simulink model "mpc_swarm_5"  (R2026a)
settings: Solver=ode4  FixedStep=0.004
undefined symbols (not defined in the file or in its folder): controlParams, eQ, eT, GravityAcc, kQ, kT, Mass, minPWM, mpc_swarm_step, rotorsSpeedDown, rotorsSpeedUp, SampleTime, uavParam
libraries: slpidlib x120, simulink x55, robotcorelib x20, matrix_library x20, aerolibasang x20, aerolibobsolete x5, uavutilslib x5
(part 5 of 14)

== system mpc_swarm_5/drone_1/pid_velocity/Subsystem ==
  roll_des : Inport
  pitch_des : Inport  Port=2
  yaw_des : Inport  Port=3
  euler_act : Inport  Port=4
  "[pqr_act" : Inport  Port=5
  Constant24 : Constant  Value=2
  Constant25 : Constant  Value=2
  Constant26 : Constant  Value=3
  Constant27 : Constant  Value=3
  Constant{30..31,35..36,42} (5 alike) : Constant  Value=0.01
  Constant32 : Constant  Value=10
  Constant33 : Constant
  Constant34 : Constant  Value=3
  Constant38 : Constant  Value=10
  Constant39 : Constant
  Constant40 : Constant  Value=5
  Constant41 : Constant  Value=0.1
  Constant49 : Constant  Value=10
  Constant50 : Constant  Value=2
  Constant7 : Constant  Value=0  OutDataTypeStr=boolean
  Demux1 : Demux  Outputs=3
  Demux5 : Demux  Outputs=3
  Gain10 : Gain  Gain=-1
  Gain11 : Gain  Gain=-1
  Gain9 : Gain  Gain=-1
  Mux : Mux  Inputs=3
  Mux4 : Mux  Inputs=3
  PID Controller3 : slpidlib/PID Controller  Controller=P  Form=Parallel  TimeDomain=Discrete-time  UseExternalTs=off  SampleTime=-1  IntegratorMethod=Forward Euler  FilterMethod=Forward Euler  ControllerParametersSource=external  P=6  I=1  UseKiTs=off  D=0.2  UseExternalDerivativeSource=off  N=100  UseFilter=on  TunerSelectOption=Transfer Function Based (PID Tuner App)  InitialConditionSource=internal  InitialConditionForIntegrator=0  InitialConditionForFilter=0  DifferentiatorICPrevScaledInput=0  ExternalReset=none  TrackingMode=off  Kt=1  LimitOutput=off  SatLimitsSource=internal  UpperSaturationLimit=inf  LowerSaturationLimit=-inf  LinearizeAsGain=on  AntiWindupMode=none  Kb=1  LimitIntegrator=off  UpperIntegratorSaturationLimit=inf  LowerIntegratorSaturationLimit=-inf  POutMin=[]  POutMax=[]  IOutMin=[]  IOutMax=[]  DOutMin=[]  DOutMax=[]  NOutMin=[]  NOutMax=[]  SumOutMin=[]  SumOutMax=[]  SaturationOutMin=[]  SaturationOutMax=[]  PParamMin=[]  PParamMax=[]  IParamMin=[]  IParamMax=[]  DParamMin=[]  DParamMax=[]  NParamMin=[]  NParamMax=[]  KbParamMin=[]  KbParamMax=[]  KtParamMin=[]  KtParamMax=[]  KbOutMin=[]  KbOutMax=[]  KtOutMin=[]  KtOutMax=[]  IntegratorOutMin=[]  IntegratorOutMax=[]  FilterOutMin=[]  FilterOutMax=[]  SumI1OutMin=[]  SumI1OutMax=[]  SumI2OutMin=[]  SumI2OutMax=[]  SumI3OutMin=[]  SumI3OutMax=[]  SumI4OutMin=[]  SumI4OutMax=[]  SumDOutMin=[]  SumDOutMax=[]  DifferentiatorOutMin=[]  DifferentiatorOutMax=[]  FilterDiffOutCoefMin=[]  FilterDiffOutCoefMax=[]  ReciprocalOutMin=[]  ReciprocalOutMax=[]  SumDenOutMin=[]  SumDenOutMax=[]  SumNumOutMin=[]  SumNumOutMax=[]  DivideOutMin=[]  DivideOutMax=[]  UdiffTsProdOutMin=[]  UdiffTsProdOutMax=[]  NTsProdOutMin=[]  NTsProdOutMax=[]  UintegralTsProdOutMin=[]  UintegralTsProdOutMax=[]  UngainTsProdOutMin=[]  UngainTsProdOutMax=[]  ClampingZeroOutDataTypeStr=Inherit: Inherit via back propagation  ClampingZeroOutMin=[]  ClampingZeroOutMax=[]  FilterDenConstantOutDataTypeStr=Inherit: Inherit via back propagation  FilterDenConstantOutMin=[]  FilterDenConstantOutMax=[]  PCopyOutDataTypeStr=Inherit: Inherit via back propagation  PCopyOutMin=[]  PCopyOutMax=[]  NCopyOutDataTypeStr=Inherit: Inherit via back propagation  NCopyOutMin=[]  NCopyOutMax=[]  IntegratorContinuousStateAttributes=''  IntegratorStateMustResolveToSignalObject=off  IntegratorRTWStateStorageClass=Auto  FilterContinuousStateAttributes=''  FilterStateMustResolveToSignalObject=off  FilterRTWStateStorageClass=Auto  ParallelPVariant=ExternalParameters  IdealPVariant=Disabled  IVariant=Disabled  DVariant=Disabled  IntegratorVariant=Disabled  SatVariant=Disabled  AWVariant=Disabled  PCopyVariant=Disabled  TRVariant=Disabled  FdbkBlocksVariant=Forward  IdealPFdbkVariant=Disabled  SatFdbkVariant=Disabled  DerivativeFilterVariant=Disabled  NVariant=Disabled  NCopyVariant=Disabled_SignalSpec  FilterICVariant=Disabled  IntegratorICVariant=Disabled  ExternalResetVariant=Disabled  TRSumVariant=Passthrough  SumFdbkVariant=Disabled  SumVariant=Passthrough_P  TsampFilterVariant=InternalTs  TsampNgainVariant=Passthrough  TsampIntegralVariant=Disabled_SignalSpec  ExternalSaturationOutDataTypeStr=Inherit: Same as second input  DerivativeSourceVariant=Disabled  PreIntVariant=InternalPreInt
  PID Controller4 : slpidlib/PID Controller  Controller=P  Form=Parallel  TimeDomain=Discrete-time  UseExternalTs=off  SampleTime=-1  IntegratorMethod=Forward Euler  FilterMethod=Forward Euler  ControllerParametersSource=external  P=5  I=1  UseKiTs=off  D=0.2  UseExternalDerivativeSource=off  N=100  UseFilter=on  TunerSelectOption=Transfer Function Based (PID Tuner App)  InitialConditionSource=internal  InitialConditionForIntegrator=0  InitialConditionForFilter=0  DifferentiatorICPrevScaledInput=0  ExternalReset=none  TrackingMode=off  Kt=1  LimitOutput=off  SatLimitsSource=internal  UpperSaturationLimit=inf  LowerSaturationLimit=-inf  LinearizeAsGain=on  AntiWindupMode=none  Kb=1  LimitIntegrator=off  UpperIntegratorSaturationLimit=inf  LowerIntegratorSaturationLimit=-inf  POutMin=[]  POutMax=[]  IOutMin=[]  IOutMax=[]  DOutMin=[]  DOutMax=[]  NOutMin=[]  NOutMax=[]  SumOutMin=[]  SumOutMax=[]  SaturationOutMin=[]  SaturationOutMax=[]  PParamMin=[]  PParamMax=[]  IParamMin=[]  IParamMax=[]  DParamMin=[]  DParamMax=[]  NParamMin=[]  NParamMax=[]  KbParamMin=[]  KbParamMax=[]  KtParamMin=[]  KtParamMax=[]  KbOutMin=[]  KbOutMax=[]  KtOutMin=[]  KtOutMax=[]  IntegratorOutMin=[]  IntegratorOutMax=[]  FilterOutMin=[]  FilterOutMax=[]  SumI1OutMin=[]  SumI1OutMax=[]  SumI2OutMin=[]  SumI2OutMax=[]  SumI3OutMin=[]  SumI3OutMax=[]  SumI4OutMin=[]  SumI4OutMax=[]  SumDOutMin=[]  SumDOutMax=[]  DifferentiatorOutMin=[]  DifferentiatorOutMax=[]  FilterDiffOutCoefMin=[]  FilterDiffOutCoefMax=[]  ReciprocalOutMin=[]  ReciprocalOutMax=[]  SumDenOutMin=[]  SumDenOutMax=[]  SumNumOutMin=[]  SumNumOutMax=[]  DivideOutMin=[]  DivideOutMax=[]  UdiffTsProdOutMin=[]  UdiffTsProdOutMax=[]  NTsProdOutMin=[]  NTsProdOutMax=[]  UintegralTsProdOutMin=[]  UintegralTsProdOutMax=[]  UngainTsProdOutMin=[]  UngainTsProdOutMax=[]  ClampingZeroOutDataTypeStr=Inherit: Inherit via back propagation  ClampingZeroOutMin=[]  ClampingZeroOutMax=[]  FilterDenConstantOutDataTypeStr=Inherit: Inherit via back propagation  FilterDenConstantOutMin=[]  FilterDenConstantOutMax=[]  PCopyOutDataTypeStr=Inherit: Inherit via back propagation  PCopyOutMin=[]  PCopyOutMax=[]  NCopyOutDataTypeStr=Inherit: Inherit via back propagation  NCopyOutMin=[]  NCopyOutMax=[]  IntegratorContinuousStateAttributes=''  IntegratorStateMustResolveToSignalObject=off  IntegratorRTWStateStorageClass=Auto  FilterContinuousStateAttributes=''  FilterStateMustResolveToSignalObject=off  FilterRTWStateStorageClass=Auto  ParallelPVariant=ExternalParameters  IdealPVariant=Disabled  IVariant=Disabled  DVariant=Disabled  IntegratorVariant=Disabled  SatVariant=Disabled  AWVariant=Disabled  PCopyVariant=Disabled  TRVariant=Disabled  FdbkBlocksVariant=Forward  IdealPFdbkVariant=Disabled  SatFdbkVariant=Disabled  DerivativeFilterVariant=Disabled  NVariant=Disabled  NCopyVariant=Disabled_SignalSpec  FilterICVariant=Disabled  IntegratorICVariant=Disabled  ExternalResetVariant=Disabled  TRSumVariant=Passthrough  SumFdbkVariant=Disabled  SumVariant=Passthrough_P  TsampFilterVariant=InternalTs  TsampNgainVariant=Passthrough  TsampIntegralVariant=Disabled_SignalSpec  ExternalSaturationOutDataTypeStr=Inherit: Same as second input  DerivativeSourceVariant=Disabled  PreIntVariant=InternalPreInt
  PID Controller5 : slpidlib/PID Controller  Controller=P  Form=Parallel  TimeDomain=Discrete-time  UseExternalTs=off  SampleTime=-1  IntegratorMethod=Forward Euler  FilterMethod=Forward Euler  ControllerParametersSource=external  P=3  I=0.0593544486366272  UseKiTs=off  D=12.4048497936965  UseExternalDerivativeSource=off  N=6.75214061700394  UseFilter=on  TunerSelectOption=Transfer Function Based (PID Tuner App)  InitialConditionSource=internal  InitialConditionForIntegrator=0  InitialConditionForFilter=0  DifferentiatorICPrevScaledInput=0  ExternalReset=none  TrackingMode=off  Kt=1  LimitOutput=off  SatLimitsSource=internal  UpperSaturationLimit=inf  LowerSaturationLimit=-inf  LinearizeAsGain=on  AntiWindupMode=none  Kb=1  LimitIntegrator=off  UpperIntegratorSaturationLimit=inf  LowerIntegratorSaturationLimit=-inf  POutMin=[]  POutMax=[]  IOutMin=[]  IOutMax=[]  DOutMin=[]  DOutMax=[]  NOutMin=[]  NOutMax=[]  SumOutMin=[]  SumOutMax=[]  SaturationOutMin=[]  SaturationOutMax=[]  PParamMin=[]  PParamMax=[]  IParamMin=[]  IParamMax=[]  DParamMin=[]  DParamMax=[]  NParamMin=[]  NParamMax=[]  KbParamMin=[]  KbParamMax=[]  KtParamMin=[]  KtParamMax=[]  KbOutMin=[]  KbOutMax=[]  KtOutMin=[]  KtOutMax=[]  IntegratorOutMin=[]  IntegratorOutMax=[]  FilterOutMin=[]  FilterOutMax=[]  SumI1OutMin=[]  SumI1OutMax=[]  SumI2OutMin=[]  SumI2OutMax=[]  SumI3OutMin=[]  SumI3OutMax=[]  SumI4OutMin=[]  SumI4OutMax=[]  SumDOutMin=[]  SumDOutMax=[]  DifferentiatorOutMin=[]  DifferentiatorOutMax=[]  FilterDiffOutCoefMin=[]  FilterDiffOutCoefMax=[]  ReciprocalOutMin=[]  ReciprocalOutMax=[]  SumDenOutMin=[]  SumDenOutMax=[]  SumNumOutMin=[]  SumNumOutMax=[]  DivideOutMin=[]  DivideOutMax=[]  UdiffTsProdOutMin=[]  UdiffTsProdOutMax=[]  NTsProdOutMin=[]  NTsProdOutMax=[]  UintegralTsProdOutMin=[]  UintegralTsProdOutMax=[]  UngainTsProdOutMin=[]  UngainTsProdOutMax=[]  ClampingZeroOutDataTypeStr=Inherit: Inherit via back propagation  ClampingZeroOutMin=[]  ClampingZeroOutMax=[]  FilterDenConstantOutDataTypeStr=Inherit: Inherit via back propagation  FilterDenConstantOutMin=[]  FilterDenConstantOutMax=[]  PCopyOutDataTypeStr=Inherit: Inherit via back propagation  PCopyOutMin=[]  PCopyOutMax=[]  NCopyOutDataTypeStr=Inherit: Inherit via back propagation  NCopyOutMin=[]  NCopyOutMax=[]  IntegratorContinuousStateAttributes=''  IntegratorStateMustResolveToSignalObject=off  IntegratorRTWStateStorageClass=Auto  FilterContinuousStateAttributes=''  FilterStateMustResolveToSignalObject=off  FilterRTWStateStorageClass=Auto  ParallelPVariant=ExternalParameters  IdealPVariant=Disabled  IVariant=Disabled  DVariant=Disabled  IntegratorVariant=Disabled  SatVariant=Disabled  AWVariant=Disabled  PCopyVariant=Disabled  TRVariant=Disabled  FdbkBlocksVariant=Forward  IdealPFdbkVariant=Disabled  SatFdbkVariant=Disabled  DerivativeFilterVariant=Disabled  NVariant=Disabled  NCopyVariant=Disabled_SignalSpec  FilterICVariant=Disabled  IntegratorICVariant=Disabled  ExternalResetVariant=Disabled  TRSumVariant=Passthrough  SumFdbkVariant=Disabled  SumVariant=Passthrough_P  TsampFilterVariant=InternalTs  TsampNgainVariant=Passthrough  TsampIntegralVariant=Disabled_SignalSpec  ExternalSaturationOutDataTypeStr=Inherit: Same as second input  DerivativeSourceVariant=Disabled  PreIntVariant=InternalPreInt
  Sum : Sum  Inputs=|+-
  Sum1 : Sum  Inputs=|+-
  Sum2 : Sum  Inputs=|+-
  pid : Subsystem
  pid1 : Subsystem
  pid2 : Subsystem
  姿态角误差 : MATLAB Function  TreatAsAtomicUnit=on
  w_phi : Outport
  w_theta : Outport  Port=2
  w_psi : Outport  Port=3
  wires:
  Mux/1 -> ?
  Sum/1 -> pid/1(u)
  Mux4/1 -> 姿态角误差/1(angle_des)  "target_att"
  Constant7/1 -> pid2/8(Reset1), pid/8(Reset1), pid1/8(Reset1)
  Constant39/1 -> pid1/6(up), Gain10/1
  Constant34/1 -> pid1/2(kP)
  Constant25/1 -> PID Controller4/2
  Sum2/1 -> pid2/1(u)
  Demux5/2 -> PID Controller4/1
  PID Controller5/1 -> Mux/3, Sum2/1
  Constant50/1 -> Gain11/1, pid2/6(up)
  euler_act/1 -> 姿态角误差/2(angle_meas)
  PID Controller4/1 -> Mux/2, Sum1/1
  Constant42/1 -> pid2/4(kD)
  Gain10/1 -> pid1/7(lo)
  yaw_des/1 -> Mux4/3
  Constant40/1 -> pid2/2(kP)
  PID Controller3/1 -> Mux/1, Sum/1
  Demux1/3 -> Sum2/2
  Constant26/1 -> PID Controller5/2
  Constant38/1 -> pid1/5(kN)
  Constant41/1 -> pid2/3(kI)
  roll_des/1 -> Mux4/1
  Constant24/1 -> PID Controller3/2
  Constant33/1 -> Gain9/1, pid/6(up)
  Demux5/3 -> PID Controller5/1
  Gain9/1 -> pid/7(lo)
  Gain11/1 -> pid2/7(lo)
  "[pqr_act"/1 -> Demux1/1
  Constant49/1 -> pid2/5(kN)
  Constant36/1 -> pid1/4(kD)
  Constant27/1 -> pid/2(kP)
  pitch_des/1 -> Mux4/2
  pid1/1(output) -> w_theta/1  "w_theta"
  Demux1/2 -> Sum1/2
  Constant30/1 -> pid/3(kI)
  Constant35/1 -> pid1/3(kI)
  pid2/1(output) -> w_psi/1  "w_psi"
  pid/1(output) -> w_phi/1  "w_phi"
  Demux1/1 -> Sum/2
  姿态角误差/1(angle_err) -> Demux5/1  "attE"
  Demux5/1 -> PID Controller3/1
  Constant31/1 -> pid/4(kD)
  Sum1/1 -> pid1/1(u)
  Constant32/1 -> pid/5(kN)

== system mpc_swarm_5/drone_1/pid_velocity/Subsystem1 ==
  zact : Inport
  zcmd : Inport  Port=2
  vzact : Inport  Port=3
  mg1_4 : Inport  Port=4
  Add : Sum  Inputs=+-
  Constant : Constant  Value=0  OutDataTypeStr=double
  Constant16 : Constant  Value=0.03  OutDataTypeStr=double
  Constant17 : Constant  Value=30  OutDataTypeStr=double
  Constant45 : Constant  Value=0  OutDataTypeStr=double
  Constant46 : Constant  Value=0  OutDataTypeStr=double
  Constant47 : Constant  OutDataTypeStr=double
  Constant9 : Constant  Value=2
  Display5 : Display
  Gain2 : Gain
  Gain4 : Gain
  PID Controller1 : slpidlib/PID Controller  Controller=P  Form=Parallel  TimeDomain=Discrete-time  UseExternalTs=off  SampleTime=-1  IntegratorMethod=Forward Euler  FilterMethod=Forward Euler  ControllerParametersSource=external  P=6  I=1  UseKiTs=off  D=0.2  UseExternalDerivativeSource=off  N=100  UseFilter=on  TunerSelectOption=Transfer Function Based (PID Tuner App)  InitialConditionSource=internal  InitialConditionForIntegrator=0  InitialConditionForFilter=0  DifferentiatorICPrevScaledInput=0  ExternalReset=none  TrackingMode=off  Kt=1  LimitOutput=off  SatLimitsSource=internal  UpperSaturationLimit=inf  LowerSaturationLimit=-inf  LinearizeAsGain=on  AntiWindupMode=none  Kb=1  LimitIntegrator=off  UpperIntegratorSaturationLimit=inf  LowerIntegratorSaturationLimit=-inf  POutMin=[]  POutMax=[]  IOutMin=[]  IOutMax=[]  DOutMin=[]  DOutMax=[]  NOutMin=[]  NOutMax=[]  SumOutMin=[]  SumOutMax=[]  SaturationOutMin=[]  SaturationOutMax=[]  PParamMin=[]  PParamMax=[]  IParamMin=[]  IParamMax=[]  DParamMin=[]  DParamMax=[]  NParamMin=[]  NParamMax=[]  KbParamMin=[]  KbParamMax=[]  KtParamMin=[]  KtParamMax=[]  KbOutMin=[]  KbOutMax=[]  KtOutMin=[]  KtOutMax=[]  IntegratorOutMin=[]  IntegratorOutMax=[]  FilterOutMin=[]  FilterOutMax=[]  SumI1OutMin=[]  SumI1OutMax=[]  SumI2OutMin=[]  SumI2OutMax=[]  SumI3OutMin=[]  SumI3OutMax=[]  SumI4OutMin=[]  SumI4OutMax=[]  SumDOutMin=[]  SumDOutMax=[]  DifferentiatorOutMin=[]  DifferentiatorOutMax=[]  FilterDiffOutCoefMin=[]  FilterDiffOutCoefMax=[]  ReciprocalOutMin=[]  ReciprocalOutMax=[]  SumDenOutMin=[]  SumDenOutMax=[]  SumNumOutMin=[]  SumNumOutMax=[]  DivideOutMin=[]  DivideOutMax=[]  UdiffTsProdOutMin=[]  UdiffTsProdOutMax=[]  NTsProdOutMin=[]  NTsProdOutMax=[]  UintegralTsProdOutMin=[]  UintegralTsProdOutMax=[]  UngainTsProdOutMin=[]  UngainTsProdOutMax=[]  ClampingZeroOutDataTypeStr=Inherit: Inherit via back propagation  ClampingZeroOutMin=[]  ClampingZeroOutMax=[]  FilterDenConstantOutDataTypeStr=Inherit: Inherit via back propagation  FilterDenConstantOutMin=[]  FilterDenConstantOutMax=[]  PCopyOutDataTypeStr=Inherit: Inherit via back propagation  PCopyOutMin=[]  PCopyOutMax=[]  NCopyOutDataTypeStr=Inherit: Inherit via back propagation  NCopyOutMin=[]  NCopyOutMax=[]  IntegratorContinuousStateAttributes=''  IntegratorStateMustResolveToSignalObject=off  IntegratorRTWStateStorageClass=Auto  FilterContinuousStateAttributes=''  FilterStateMustResolveToSignalObject=off  FilterRTWStateStorageClass=Auto  ParallelPVariant=ExternalParameters  IdealPVariant=Disabled  IVariant=Disabled  DVariant=Disabled  IntegratorVariant=Disabled  SatVariant=Disabled  AWVariant=Disabled  PCopyVariant=Disabled  TRVariant=Disabled  FdbkBlocksVariant=Forward  IdealPFdbkVariant=Disabled  SatFdbkVariant=Disabled  DerivativeFilterVariant=Disabled  NVariant=Disabled  NCopyVariant=Disabled_SignalSpec  FilterICVariant=Disabled  IntegratorICVariant=Disabled  ExternalResetVariant=Disabled  TRSumVariant=Passthrough  SumFdbkVariant=Disabled  SumVariant=Passthrough_P  TsampFilterVariant=InternalTs  TsampNgainVariant=Passthrough  TsampIntegralVariant=Disabled_SignalSpec  ExternalSaturationOutDataTypeStr=Inherit: Same as second input  DerivativeSourceVariant=Disabled  PreIntVariant=InternalPreInt
  Saturation8 : Saturate  UpperLimit=2  LowerLimit=-2
  Sum3 : Sum  Inputs=|-+
  pid3 : Subsystem
  w_z : Outport
  wires:
  Constant47/1 -> pid3/8(Reset1)
  Constant/1 -> pid3/3(kI)
  vzact/1 -> Gain4/1
  Constant45/1 -> pid3/6(up)
  Gain4/1 -> Sum3/2
  Constant46/1 -> pid3/7(lo)
  Saturation8/1 -> Sum3/1
  Constant16/1 -> pid3/4(kD)
  Constant17/1 -> pid3/5(kN)
  PID Controller1/1 -> Saturation8/1  "w_z"
  Sum3/1 -> pid3/1(u)
  zact/1 -> Add/1
  zcmd/1 -> Gain2/1
  Constant9/1 -> PID Controller1/2
  Add/1 -> Display5/1, PID Controller1/1
  Gain2/1 -> Add/2
  pid3/1(output) -> w_z/1  "w_z"
  mg1_4/1 -> pid3/2(kP)

== system mpc_swarm_5/drone_1/pid_velocity/水平和高度控制 ==
  note: 该位置控制器，参考全权文献中的11.3.2的2.开源自驾仪中的pid控制器的相关内容
  vxyz_des : Inport
  euler_act : Inport  Port=2
  pos_act : Inport  Port=3
  v_act : Inport  Port=4
  mg1_4 : Inport  Port=5
  Constant : Constant  Value=0
  Demux{,1..3} (4 alike) : Demux  Outputs=3
  Gain2 : Gain  Gain=180/pi
  MATLAB Function : MATLAB Function  TreatAsAtomicUnit=on
  PID Controller : slpidlib/PID Controller  Controller=P  Form=Parallel  TimeDomain=Continuous-time  UseExternalTs=off  SampleTime=-1  IntegratorMethod=Forward Euler  FilterMethod=Forward Euler  ControllerParametersSource=internal  P=1  I=0  UseKiTs=off  D=0  UseExternalDerivativeSource=off  N=100  UseFilter=on  TunerSelectOption=Transfer Function Based (PID Tuner App)  InitialConditionSource=internal  InitialConditionForIntegrator=0  InitialConditionForFilter=0  DifferentiatorICPrevScaledInput=0  ExternalReset=none  TrackingMode=off  Kt=1  LimitOutput=off  SatLimitsSource=internal  UpperSaturationLimit=inf  LowerSaturationLimit=-inf  LinearizeAsGain=on  AntiWindupMode=none  Kb=1  LimitIntegrator=off  UpperIntegratorSaturationLimit=inf  LowerIntegratorSaturationLimit=-inf  POutMin=[]  POutMax=[]  IOutMin=[]  IOutMax=[]  DOutMin=[]  DOutMax=[]  NOutMin=[]  NOutMax=[]  SumOutMin=[]  SumOutMax=[]  SaturationOutMin=[]  SaturationOutMax=[]  PParamMin=[]  PParamMax=[]  IParamMin=[]  IParamMax=[]  DParamMin=[]  DParamMax=[]  NParamMin=[]  NParamMax=[]  KbParamMin=[]  KbParamMax=[]  KtParamMin=[]  KtParamMax=[]  KbOutMin=[]  KbOutMax=[]  KtOutMin=[]  KtOutMax=[]  IntegratorOutMin=[]  IntegratorOutMax=[]  FilterOutMin=[]  FilterOutMax=[]  SumI1OutMin=[]  SumI1OutMax=[]  SumI2OutMin=[]  SumI2OutMax=[]  SumI3OutMin=[]  SumI3OutMax=[]  SumI4OutMin=[]  SumI4OutMax=[]  SumDOutMin=[]  SumDOutMax=[]  DifferentiatorOutMin=[]  DifferentiatorOutMax=[]  FilterDiffOutCoefMin=[]  FilterDiffOutCoefMax=[]  ReciprocalOutMin=[]  ReciprocalOutMax=[]  SumDenOutMin=[]  SumDenOutMax=[]  SumNumOutMin=[]  SumNumOutMax=[]  DivideOutMin=[]  DivideOutMax=[]  UdiffTsProdOutMin=[]  UdiffTsProdOutMax=[]  NTsProdOutMin=[]  NTsProdOutMax=[]  UintegralTsProdOutMin=[]  UintegralTsProdOutMax=[]  UngainTsProdOutMin=[]  UngainTsProdOutMax=[]  ClampingZeroOutDataTypeStr=Inherit: Inherit via back propagation  ClampingZeroOutMin=[]  ClampingZeroOutMax=[]  FilterDenConstantOutDataTypeStr=Inherit: Inherit via back propagation  FilterDenConstantOutMin=[]  FilterDenConstantOutMax=[]  PCopyOutDataTypeStr=Inherit: Inherit via back propagation  PCopyOutMin=[]  PCopyOutMax=[]  NCopyOutDataTypeStr=Inherit: Inherit via back propagation  NCopyOutMin=[]  NCopyOutMax=[]  IntegratorContinuousStateAttributes=''  IntegratorStateMustResolveToSignalObject=off  IntegratorRTWStateStorageClass=Auto  FilterContinuousStateAttributes=''  FilterStateMustResolveToSignalObject=off  FilterRTWStateStorageClass=Auto  ParallelPVariant=InternalParameters  IdealPVariant=Disabled  IVariant=Disabled  DVariant=Disabled  IntegratorVariant=Disabled  SatVariant=Disabled  AWVariant=Disabled  PCopyVariant=Disabled  TRVariant=Disabled  FdbkBlocksVariant=Forward  IdealPFdbkVariant=Disabled  SatFdbkVariant=Disabled  DerivativeFilterVariant=Disabled  NVariant=Disabled  NCopyVariant=Disabled_SignalSpec  FilterICVariant=Disabled  IntegratorICVariant=Disabled  ExternalResetVariant=Disabled  TRSumVariant=Passthrough  SumFdbkVariant=Disabled  SumVariant=Passthrough_P  TsampFilterVariant=InternalTs  TsampNgainVariant=Passthrough  TsampIntegralVariant=Disabled_SignalSpec  ExternalSaturationOutDataTypeStr=Inherit: Same as second input  DerivativeSourceVariant=Disabled  PreIntVariant=InternalPreInt
  PID Controller1 : slpidlib/PID Controller  Controller=PID  Form=Parallel  TimeDomain=Discrete-time  UseExternalTs=off  SampleTime=-1  IntegratorMethod=Forward Euler  FilterMethod=Forward Euler  ControllerParametersSource=internal  P=3  I=0.2  UseKiTs=off  D=0  UseExternalDerivativeSource=off  N=100  UseFilter=on  TunerSelectOption=Transfer Function Based (PID Tuner App)  InitialConditionSource=internal  InitialConditionForIntegrator=0  InitialConditionForFilter=0  DifferentiatorICPrevScaledInput=0  ExternalReset=none  TrackingMode=off  Kt=1  LimitOutput=off  SatLimitsSource=internal  UpperSaturationLimit=inf  LowerSaturationLimit=-inf  LinearizeAsGain=on  AntiWindupMode=none  Kb=1  LimitIntegrator=off  UpperIntegratorSaturationLimit=inf  LowerIntegratorSaturationLimit=-inf  POutMin=[]  POutMax=[]  IOutMin=[]  IOutMax=[]  DOutMin=[]  DOutMax=[]  NOutMin=[]  NOutMax=[]  SumOutMin=[]  SumOutMax=[]  SaturationOutMin=[]  SaturationOutMax=[]  PParamMin=[]  PParamMax=[]  IParamMin=[]  IParamMax=[]  DParamMin=[]  DParamMax=[]  NParamMin=[]  NParamMax=[]  KbParamMin=[]  KbParamMax=[]  KtParamMin=[]  KtParamMax=[]  KbOutMin=[]  KbOutMax=[]  KtOutMin=[]  KtOutMax=[]  IntegratorOutMin=[]  IntegratorOutMax=[]  FilterOutMin=[]  FilterOutMax=[]  SumI1OutMin=[]  SumI1OutMax=[]  SumI2OutMin=[]  SumI2OutMax=[]  SumI3OutMin=[]  SumI3OutMax=[]  SumI4OutMin=[]  SumI4OutMax=[]  SumDOutMin=[]  SumDOutMax=[]  DifferentiatorOutMin=[]  DifferentiatorOutMax=[]  FilterDiffOutCoefMin=[]  FilterDiffOutCoefMax=[]  ReciprocalOutMin=[]  ReciprocalOutMax=[]  SumDenOutMin=[]  SumDenOutMax=[]  SumNumOutMin=[]  SumNumOutMax=[]  DivideOutMin=[]  DivideOutMax=[]  UdiffTsProdOutMin=[]  UdiffTsProdOutMax=[]  NTsProdOutMin=[]  NTsProdOutMax=[]  UintegralTsProdOutMin=[]  UintegralTsProdOutMax=[]  UngainTsProdOutMin=[]  UngainTsProdOutMax=[]  ClampingZeroOutDataTypeStr=Inherit: Inherit via back propagation  ClampingZeroOutMin=[]  ClampingZeroOutMax=[]  FilterDenConstantOutDataTypeStr=Inherit: Inherit via back propagation  FilterDenConstantOutMin=[]  FilterDenConstantOutMax=[]  PCopyOutDataTypeStr=Inherit: Inherit via back propagation  PCopyOutMin=[]  PCopyOutMax=[]  NCopyOutDataTypeStr=Inherit: Inherit via back propagation  NCopyOutMin=[]  NCopyOutMax=[]  IntegratorContinuousStateAttributes=''  IntegratorStateMustResolveToSignalObject=off  IntegratorRTWStateStorageClass=Auto  FilterContinuousStateAttributes=''  FilterStateMustResolveToSignalObject=off  FilterRTWStateStorageClass=Auto  ParallelPVariant=InternalParameters  IdealPVariant=Disabled  IVariant=InternalParameters  DVariant=InternalParameters  IntegratorVariant=Discrete  SatVariant=Disabled  AWVariant=Passthrough  PCopyVariant=Disabled  TRVariant=Disabled  FdbkBlocksVariant=Forward  IdealPFdbkVariant=Disabled  SatFdbkVariant=Disabled  DerivativeFilterVariant=ForwardEulerFilter  NVariant=InternalParameters  NCopyVariant=Disabled  FilterICVariant=InternalICsFilter  IntegratorICVariant=InternalICs  ExternalResetVariant=Disabled  TRSumVariant=Passthrough  SumFdbkVariant=Disabled  SumVariant=Sum_PID  TsampFilterVariant=InternalTs  TsampNgainVariant=Passthrough  TsampIntegralVariant=Disabled_SignalSpec  ExternalSaturationOutDataTypeStr=Inherit: Same as second input  DerivativeSourceVariant=ErrorSignal  PreIntVariant=InternalPreInt
  PID Controller2 : slpidlib/PID Controller  Controller=PID  Form=Parallel  TimeDomain=Discrete-time  UseExternalTs=off  SampleTime=-1  IntegratorMethod=Forward Euler  FilterMethod=Forward Euler  ControllerParametersSource=internal  P=3  I=0.2  UseKiTs=off  D=0  UseExternalDerivativeSource=off  N=100  UseFilter=on  TunerSelectOption=Transfer Function Based (PID Tuner App)  InitialConditionSource=internal  InitialConditionForIntegrator=0  InitialConditionForFilter=0  DifferentiatorICPrevScaledInput=0  ExternalReset=none  TrackingMode=off  Kt=1  LimitOutput=off  SatLimitsSource=internal  UpperSaturationLimit=inf  LowerSaturationLimit=-inf  LinearizeAsGain=on  AntiWindupMode=none  Kb=1  LimitIntegrator=off  UpperIntegratorSaturationLimit=inf  LowerIntegratorSaturationLimit=-inf  POutMin=[]  POutMax=[]  IOutMin=[]  IOutMax=[]  DOutMin=[]  DOutMax=[]  NOutMin=[]  NOutMax=[]  SumOutMin=[]  SumOutMax=[]  SaturationOutMin=[]  SaturationOutMax=[]  PParamMin=[]  PParamMax=[]  IParamMin=[]  IParamMax=[]  DParamMin=[]  DParamMax=[]  NParamMin=[]  NParamMax=[]  KbParamMin=[]  KbParamMax=[]  KtParamMin=[]  KtParamMax=[]  KbOutMin=[]  KbOutMax=[]  KtOutMin=[]  KtOutMax=[]  IntegratorOutMin=[]  IntegratorOutMax=[]  FilterOutMin=[]  FilterOutMax=[]  SumI1OutMin=[]  SumI1OutMax=[]  SumI2OutMin=[]  SumI2OutMax=[]  SumI3OutMin=[]  SumI3OutMax=[]  SumI4OutMin=[]  SumI4OutMax=[]  SumDOutMin=[]  SumDOutMax=[]  DifferentiatorOutMin=[]  DifferentiatorOutMax=[]  FilterDiffOutCoefMin=[]  FilterDiffOutCoefMax=[]  ReciprocalOutMin=[]  ReciprocalOutMax=[]  SumDenOutMin=[]  SumDenOutMax=[]  SumNumOutMin=[]  SumNumOutMax=[]  DivideOutMin=[]  DivideOutMax=[]  UdiffTsProdOutMin=[]  UdiffTsProdOutMax=[]  NTsProdOutMin=[]  NTsProdOutMax=[]  UintegralTsProdOutMin=[]  UintegralTsProdOutMax=[]  UngainTsProdOutMin=[]  UngainTsProdOutMax=[]  ClampingZeroOutDataTypeStr=Inherit: Inherit via back propagation  ClampingZeroOutMin=[]  ClampingZeroOutMax=[]  FilterDenConstantOutDataTypeStr=Inherit: Inherit via back propagation  FilterDenConstantOutMin=[]  FilterDenConstantOutMax=[]  PCopyOutDataTypeStr=Inherit: Inherit via back propagation  PCopyOutMin=[]  PCopyOutMax=[]  NCopyOutDataTypeStr=Inherit: Inherit via back propagation  NCopyOutMin=[]  NCopyOutMax=[]  IntegratorContinuousStateAttributes=''  IntegratorStateMustResolveToSignalObject=off  IntegratorRTWStateStorageClass=Auto  FilterContinuousStateAttributes=''  FilterStateMustResolveToSignalObject=off  FilterRTWStateStorageClass=Auto  ParallelPVariant=InternalParameters  IdealPVariant=Disabled  IVariant=InternalParameters  DVariant=InternalParameters  IntegratorVariant=Discrete  SatVariant=Disabled  AWVariant=Passthrough  PCopyVariant=Disabled  TRVariant=Disabled  FdbkBlocksVariant=Forward  IdealPFdbkVariant=Disabled  SatFdbkVariant=Disabled  DerivativeFilterVariant=ForwardEulerFilter  NVariant=InternalParameters  NCopyVariant=Disabled  FilterICVariant=InternalICsFilter  IntegratorICVariant=InternalICs  ExternalResetVariant=Disabled  TRSumVariant=Passthrough  SumFdbkVariant=Disabled  SumVariant=Sum_PID  TsampFilterVariant=InternalTs  TsampNgainVariant=Passthrough  TsampIntegralVariant=Disabled_SignalSpec  ExternalSaturationOutDataTypeStr=Inherit: Same as second input  DerivativeSourceVariant=ErrorSignal  PreIntVariant=InternalPreInt
  PID Controller3 : slpidlib/PID Controller  Controller=P  Form=Parallel  TimeDomain=Continuous-time  UseExternalTs=off  SampleTime=-1  IntegratorMethod=Forward Euler  FilterMethod=Forward Euler  ControllerParametersSource=internal  P=1  I=0  UseKiTs=off  D=0  UseExternalDerivativeSource=off  N=100  UseFilter=on  TunerSelectOption=Transfer Function Based (PID Tuner App)  InitialConditionSource=internal  InitialConditionForIntegrator=0  InitialConditionForFilter=0  DifferentiatorICPrevScaledInput=0  ExternalReset=none  TrackingMode=off  Kt=1  LimitOutput=off  SatLimitsSource=internal  UpperSaturationLimit=inf  LowerSaturationLimit=-inf  LinearizeAsGain=on  AntiWindupMode=none  Kb=1  LimitIntegrator=off  UpperIntegratorSaturationLimit=inf  LowerIntegratorSaturationLimit=-inf  POutMin=[]  POutMax=[]  IOutMin=[]  IOutMax=[]  DOutMin=[]  DOutMax=[]  NOutMin=[]  NOutMax=[]  SumOutMin=[]  SumOutMax=[]  SaturationOutMin=[]  SaturationOutMax=[]  PParamMin=[]  PParamMax=[]  IParamMin=[]  IParamMax=[]  DParamMin=[]  DParamMax=[]  NParamMin=[]  NParamMax=[]  KbParamMin=[]  KbParamMax=[]  KtParamMin=[]  KtParamMax=[]  KbOutMin=[]  KbOutMax=[]  KtOutMin=[]  KtOutMax=[]  IntegratorOutMin=[]  IntegratorOutMax=[]  FilterOutMin=[]  FilterOutMax=[]  SumI1OutMin=[]  SumI1OutMax=[]  SumI2OutMin=[]  SumI2OutMax=[]  SumI3OutMin=[]  SumI3OutMax=[]  SumI4OutMin=[]  SumI4OutMax=[]  SumDOutMin=[]  SumDOutMax=[]  DifferentiatorOutMin=[]  DifferentiatorOutMax=[]  FilterDiffOutCoefMin=[]  FilterDiffOutCoefMax=[]  ReciprocalOutMin=[]  ReciprocalOutMax=[]  SumDenOutMin=[]  SumDenOutMax=[]  SumNumOutMin=[]  SumNumOutMax=[]  DivideOutMin=[]  DivideOutMax=[]  UdiffTsProdOutMin=[]  UdiffTsProdOutMax=[]  NTsProdOutMin=[]  NTsProdOutMax=[]  UintegralTsProdOutMin=[]  UintegralTsProdOutMax=[]  UngainTsProdOutMin=[]  UngainTsProdOutMax=[]  ClampingZeroOutDataTypeStr=Inherit: Inherit via back propagation  ClampingZeroOutMin=[]  ClampingZeroOutMax=[]  FilterDenConstantOutDataTypeStr=Inherit: Inherit via back propagation  FilterDenConstantOutMin=[]  FilterDenConstantOutMax=[]  PCopyOutDataTypeStr=Inherit: Inherit via back propagation  PCopyOutMin=[]  PCopyOutMax=[]  NCopyOutDataTypeStr=Inherit: Inherit via back propagation  NCopyOutMin=[]  NCopyOutMax=[]  IntegratorContinuousStateAttributes=''  IntegratorStateMustResolveToSignalObject=off  IntegratorRTWStateStorageClass=Auto  FilterContinuousStateAttributes=''  FilterStateMustResolveToSignalObject=off  FilterRTWStateStorageClass=Auto  ParallelPVariant=InternalParameters  IdealPVariant=Disabled  IVariant=Disabled  DVariant=Disabled  IntegratorVariant=Disabled  SatVariant=Disabled  AWVariant=Disabled  PCopyVariant=Disabled  TRVariant=Disabled  FdbkBlocksVariant=Forward  IdealPFdbkVariant=Disabled  SatFdbkVariant=Disabled  DerivativeFilterVariant=Disabled  NVariant=Disabled  NCopyVariant=Disabled_SignalSpec  FilterICVariant=Disabled  IntegratorICVariant=Disabled  ExternalResetVariant=Disabled  TRSumVariant=Passthrough  SumFdbkVariant=Disabled  SumVariant=Passthrough_P  TsampFilterVariant=InternalTs  TsampNgainVariant=Passthrough  TsampIntegralVariant=Disabled_SignalSpec  ExternalSaturationOutDataTypeStr=Inherit: Same as second input  DerivativeSourceVariant=Disabled  PreIntVariant=InternalPreInt
  Saturation : Saturate  UpperLimit=0.6  LowerLimit=-0.6
  Saturation1 : Saturate  UpperLimit=0.6  LowerLimit=-0.6
  Saturation2 : Saturate  UpperLimit=3  LowerLimit=-3
  Saturation3 : Saturate  UpperLimit=3  LowerLimit=-3
  Subsystem1 : Subsystem
  Sum{,1,3..4} (4 alike) : Sum  Inputs=|+-
  g : Constant  Value=GravityAcc
  高度控制器 : Subsystem  Commented=on
  Thrust_desire : Outport  VectorParamsAs1DForOutWhenUnconnected=off
  roll_d : Outport  Port=2  VectorParamsAs1DForOutWhenUnconnected=off
  pitch_d : Outport  Port=3  VectorParamsAs1DForOutWhenUnconnected=off
  wires:
  Saturation2/1 -> PID Controller2/1
  euler_act/1 -> Demux2/1
  pos_act/1 -> Demux/1
  Demux/2 -> Sum1/2
  Sum/1 -> PID Controller/1
  Sum1/1 -> PID Controller3/1
  Sum4/1 -> Saturation3/1
  ? -> Sum1/1
  Demux/1 -> Sum/2
  g/1 -> MATLAB Function/4(g)
  v_act/1 -> Demux1/1
  Saturation/1 -> roll_d/1
  Demux1/1 -> Sum3/2
  Saturation1/1 -> pitch_d/1
  PID Controller2/1 -> MATLAB Function/1(v_x)
  MATLAB Function/1(roll_d) -> Saturation/1
  Sum3/1 -> Saturation2/1
  PID Controller1/1 -> MATLAB Function/2(v_y)
  Demux1/2 -> Sum4/2
  Saturation3/1 -> PID Controller1/1
  ? -> Sum/1
  MATLAB Function/2(pitch_d) -> Saturation1/1
  Demux1/3 -> [vzact]  "vz_act"
  Demux/3 -> [zact]  "z_act"
  Demux2/3 -> [actyaw]  "act_yaw"
  [actyaw] -> MATLAB Function/3(act_yaw)
  Demux3/1 -> Sum3/1  "vxd"
  高度控制器/1(Thrust_d) -> ?
  [zact] -> 高度控制器/2(z_act), Subsystem1/1(zact)
  [vzact] -> 高度控制器/3(vz_act), Subsystem1/3(vzact)
  vxyz_des/1 -> Demux3/1
  Demux3/3 -> Subsystem1/2(vzcmd)  "vzd"
  Subsystem1/1(w_z) -> Thrust_desire/1
  mg1_4/1 -> Subsystem1/4(mg1_4)
  Demux3/2 -> Sum4/1  "vyd"

== system mpc_swarm_5/drone_2/Subsystem/Rotor Assembly 1 ==
  note: RotorArm1=[ 0.375 0.375 0];
  N : Inport
  Vb : Inport  Port=2
  Arm : Inport  Port=3
  Tilt : Inport  Port=4
  TurnDirection : Inport  Port=5
  Adjust Force/Moment to Body Frame : Subsystem
  Display{2,7,9..12} (6 alike) : Display
  Gain : Gain  Commented=on  Gain=2*pi
  Gain1 : Gain  Commented=on  Gain=uavParam.motor.RPMMAX/60
  "Incidence, Sideslip, & Airspeed" : aerolibasang/Incidence, Sideslip, & Airspeed
  Saturation : Saturate  Commented=on  UpperLimit=1  LowerLimit=minPWM
  Saturation2 : Saturate  UpperLimit=rotorsSpeedUp  LowerLimit=rotorsSpeedDown
  Subsystem : Subsystem
  F : Outport
  M : Outport  Port=2
  w : Outport  Port=3
  kT : Outport  Port=4
  kQ : Outport  Port=5
  wires:
  TurnDirection/1 -> Adjust Force/Moment to Body Frame/4(TurnDirection)
  Adjust Force/Moment to Body Frame/1(Fbody) -> F/1
  Vb/1 -> "Incidence, Sideslip, & Airspeed"/1
  Saturation/1 -> Gain1/1
  Gain1/1 -> Gain/1  "W"
  Tilt/1 -> Adjust Force/Moment to Body Frame/3(Tilt)
  Subsystem/1(Fxyz) -> Adjust Force/Moment to Body Frame/1(Fmotor), Display9/1
  N/1 -> Saturation2/1
  Saturation2/1 -> w/1, Display2/1, Subsystem/2(Omega)
  Arm/1 -> Adjust Force/Moment to Body Frame/5(Arm1)
  Adjust Force/Moment to Body Frame/2(Mbody) -> M/1
  Subsystem/2(Mxyz) -> Adjust Force/Moment to Body Frame/2(Mmotor), Display7/1
  "Incidence, Sideslip, & Airspeed"/3 -> Display12/1, Subsystem/1(Va)  "airspeed"
  Subsystem/3(kT) -> kT/1, Display10/1
  Subsystem/4(kQ) -> kQ/1, Display11/1

== system mpc_swarm_5/drone_2/Subsystem/Rotor Assembly 2 ==
  note: RotorArm1=[ 0.375 0.375 0];
  N : Inport
  Vb : Inport  Port=2
  Arm : Inport  Port=3
  Tilt : Inport  Port=4
  TurnDirection : Inport  Port=5
  Adjust Force/Moment to Body Frame : Subsystem
  Display{2,7,9..12} (6 alike) : Display
  Gain : Gain  Commented=on  Gain=2*pi
  Gain1 : Gain  Commented=on  Gain=uavParam.motor.RPMMAX/60
  "Incidence, Sideslip, & Airspeed" : aerolibasang/Incidence, Sideslip, & Airspeed
  Saturation : Saturate  Commented=on  UpperLimit=1  LowerLimit=minPWM
  Saturation2 : Saturate  UpperLimit=rotorsSpeedUp  LowerLimit=rotorsSpeedDown
  Subsystem : Subsystem
  F : Outport
  M : Outport  Port=2
  w : Outport  Port=3
  kT : Outport  Port=4
  kQ : Outport  Port=5
  wires:
  Subsystem/4(kQ) -> Display11/1, kQ/1
  Subsystem/3(kT) -> Display10/1, kT/1
  "Incidence, Sideslip, & Airspeed"/3 -> Subsystem/1(Va), Display12/1  "airspeed"
  Subsystem/2(Mxyz) -> Display7/1, Adjust Force/Moment to Body Frame/2(Mmotor)
  Adjust Force/Moment to Body Frame/2(Mbody) -> M/1
  Arm/1 -> Adjust Force/Moment to Body Frame/5(Arm1)
  Saturation2/1 -> Subsystem/2(Omega), Display2/1, w/1
  N/1 -> Saturation2/1
  Subsystem/1(Fxyz) -> Display9/1, Adjust Force/Moment to Body Frame/1(Fmotor)
  Tilt/1 -> Adjust Force/Moment to Body Frame/3(Tilt)
  Gain1/1 -> Gain/1  "W"
  Saturation/1 -> Gain1/1
  Vb/1 -> "Incidence, Sideslip, & Airspeed"/1
  Adjust Force/Moment to Body Frame/1(Fbody) -> F/1
  TurnDirection/1 -> Adjust Force/Moment to Body Frame/4(TurnDirection)

== system mpc_swarm_5/drone_2/Subsystem/Rotor Assembly 3 ==
  note: RotorArm1=[ 0.375 0.375 0];
  N : Inport
  Vb : Inport  Port=2
  Arm : Inport  Port=3
  Tilt : Inport  Port=4
  TurnDirection : Inport  Port=5
  Adjust Force/Moment to Body Frame : Subsystem
  Display{2,7,9..12} (6 alike) : Display
  Gain : Gain  Commented=on  Gain=2*pi
  Gain1 : Gain  Commented=on  Gain=uavParam.motor.RPMMAX/60
  "Incidence, Sideslip, & Airspeed" : aerolibasang/Incidence, Sideslip, & Airspeed
  Saturation : Saturate  Commented=on  UpperLimit=1  LowerLimit=minPWM
  Saturation2 : Saturate  UpperLimit=rotorsSpeedUp  LowerLimit=rotorsSpeedDown
  Subsystem : Subsystem
  F : Outport
  M : Outport  Port=2
  w : Outport  Port=3
  kT : Outport  Port=4
  kQ : Outport  Port=5
  wires:
  Subsystem/4(kQ) -> Display11/1, kQ/1
  Subsystem/3(kT) -> Display10/1, kT/1
  "Incidence, Sideslip, & Airspeed"/3 -> Subsystem/1(Va), Display12/1  "airspeed"
  Subsystem/2(Mxyz) -> Display7/1, Adjust Force/Moment to Body Frame/2(Mmotor)
  Adjust Force/Moment to Body Frame/2(Mbody) -> M/1
  Arm/1 -> Adjust Force/Moment to Body Frame/5(Arm1)
  Saturation2/1 -> Subsystem/2(Omega), Display2/1, w/1
  N/1 -> Saturation2/1
  Subsystem/1(Fxyz) -> Display9/1, Adjust Force/Moment to Body Frame/1(Fmotor)
  Tilt/1 -> Adjust Force/Moment to Body Frame/3(Tilt)
  Gain1/1 -> Gain/1  "W"
  Saturation/1 -> Gain1/1
  Vb/1 -> "Incidence, Sideslip, & Airspeed"/1
  Adjust Force/Moment to Body Frame/1(Fbody) -> F/1
  TurnDirection/1 -> Adjust Force/Moment to Body Frame/4(TurnDirection)

== system mpc_swarm_5/drone_2/Subsystem/Rotor Assembly 4 ==
  note: RotorArm1=[ 0.375 0.375 0];
  N : Inport
  Vb : Inport  Port=2
  Arm : Inport  Port=3
  Tilt : Inport  Port=4
  TurnDirection : Inport  Port=5
  Adjust Force/Moment to Body Frame : Subsystem
  Display{2,7,9..12} (6 alike) : Display
  Gain : Gain  Commented=on  Gain=2*pi
  Gain1 : Gain  Commented=on  Gain=uavParam.motor.RPMMAX/60
  "Incidence, Sideslip, & Airspeed" : aerolibasang/Incidence, Sideslip, & Airspeed
  Saturation : Saturate  Commented=on  UpperLimit=1  LowerLimit=minPWM
  Saturation2 : Saturate  UpperLimit=rotorsSpeedUp  LowerLimit=rotorsSpeedDown
  Subsystem : Subsystem
  F : Outport
  M : Outport  Port=2
  w : Outport  Port=3
  kT : Outport  Port=4
  kQ : Outport  Port=5
  wires:
  TurnDirection/1 -> Adjust Force/Moment to Body Frame/4(TurnDirection)
  Adjust Force/Moment to Body Frame/1(Fbody) -> F/1
  Vb/1 -> "Incidence, Sideslip, & Airspeed"/1
  Saturation/1 -> Gain1/1
  Gain1/1 -> Gain/1  "W"
  Tilt/1 -> Adjust Force/Moment to Body Frame/3(Tilt)
  Subsystem/1(Fxyz) -> Adjust Force/Moment to Body Frame/1(Fmotor), Display9/1
  N/1 -> Saturation2/1
  Saturation2/1 -> w/1, Display2/1, Subsystem/2(Omega)
  Arm/1 -> Adjust Force/Moment to Body Frame/5(Arm1)
  Adjust Force/Moment to Body Frame/2(Mbody) -> M/1
  Subsystem/2(Mxyz) -> Adjust Force/Moment to Body Frame/2(Mmotor), Display7/1
  "Incidence, Sideslip, & Airspeed"/3 -> Display12/1, Subsystem/1(Va)  "airspeed"
  Subsystem/3(kT) -> kT/1, Display10/1
  Subsystem/4(kQ) -> kQ/1, Display11/1

== system mpc_swarm_5/drone_2/pid_velocity/Forward position ==
  e_y : Inport
  e_x : Inport  Port=2
  sin : Inport  Port=3
  cos : Inport  Port=4
  Add : Sum
  Product : Product
  Product1 : Product
  ef : Outport
  wires:
  cos/1 -> Product/1
  sin/1 -> Product1/2
  e_y/1 -> Product1/1
  e_x/1 -> Product/2
  Product/1 -> Add/1
  Product1/1 -> Add/2
  Add/1 -> ef/1

== system mpc_swarm_5/drone_2/pid_velocity/Forward velocity ==
  vy : Inport
  vx : Inport  Port=2
  sin : Inport  Port=3
  cos : Inport  Port=4
  Add : Sum
  Product : Product
  Product1 : Product
  ef : Outport
  wires:
  Add/1 -> ef/1
  Product1/1 -> Add/2
  Product/1 -> Add/1
  vx/1 -> Product/2
  vy/1 -> Product1/1
  sin/1 -> Product1/2
  cos/1 -> Product/1

== system mpc_swarm_5/drone_2/pid_velocity/Lateral position ==
  e_y : Inport
  e_x : Inport  Port=2
  sin : Inport  Port=3
  cos : Inport  Port=4
  Add : Sum
  Gain : Gain  Gain=-1
  Product : Product
  Product1 : Product
  el : Outport
  wires:
  Gain/1 -> Add/1
  Add/1 -> el/1
  Product1/1 -> Add/2
  Product/1 -> Gain/1
  cos/1 -> Product1/2
  sin/1 -> Product/1
  e_x/1 -> Product/2
  e_y/1 -> Product1/1

== system mpc_swarm_5/drone_2/pid_velocity/Lateral velocity ==
  vy : Inport
  vx : Inport  Port=2
  sin : Inport  Port=3
  cos : Inport  Port=4
  Add : Sum
  Gain : Gain  Gain=-1
  Product : Product
  Product1 : Product
  el : Outport
  wires:
  vy/1 -> Product1/1
  vx/1 -> Product/2
  sin/1 -> Product/1
  cos/1 -> Product1/2
  Product/1 -> Gain/1
  Product1/1 -> Add/2
  Add/1 -> el/1
  Gain/1 -> Add/1
